simulink model "basicLineFollowing"  (R2016b)
settings: Solver=FixedStepAuto  StartTime=0.0  StopTime=10.0  RelTol=1e-3  EnableMultiTasking=on
undefined symbols (not defined in the file): Comp, Int
libraries: legoev3lib x5
settings Model: ExtModeTrigDuration=2  Creator=Nexel  LastModifiedBy=Nexel
settings SolverCC: PositivePriorityOrder=on
settings OptimizationCC: MaxStackSize=64
settings DebuggingCC: ParameterTunabilityLossMsg=error
settings HardwareCC: ProdBitPerPointer=32  ProdBitPerSizeT=32  ProdBitPerPtrDiffT=32  ProdLargestAtomicInteger=Long  ProdWordSize=32  ProdHWDeviceType=ARM Compatible->ARM 9
settings RTWCC: SystemTargetFile=ert.tlc  HardwareBoard=LEGO MINDSTORMS EV3  TLCOptions="-aInlineSetEventsForThisBaseRateFcn=TLC_FALSE -aSuppressMultiTaskScheduler=TLC_FALSE  -aRateBasedStepFcn=0"  TemplateMakefile=ert_default_tmf  Description=Embedded Coder  GenerateReport=on  Toolchain=Sourcery G++ Lite v2009q3  IncludeHyperlinkInReport=on  LaunchReport=on  GenerateTraceInfo=on  GenerateTraceReport=on  GenerateTraceReportSl=on  GenerateTraceReportSf=on  GenerateTraceReportEml=on
settings CodeAppCC: ForceParamTrailComments=on  IgnoreCustomStorageClasses=off  OperatorAnnotations=on  SimulinkDataObjDesc=on  SFDataObjDesc=on  MATLABFcnDesc=on  InsertBlockDesc=on  MATLABSourceComments=on
settings ERTTargetCC: SupportContinuousTime=on  SupportVariableSizeSignals=on

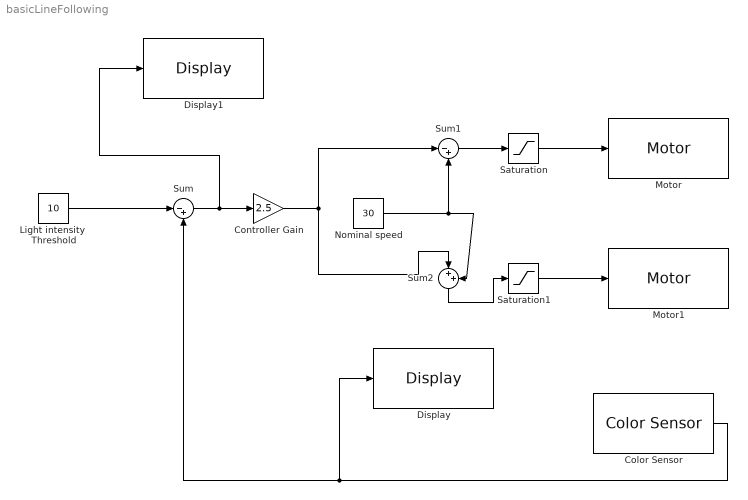
== system basicLineFollowing ==
  Color Sensor : legoev3lib/Color Sensor  portNumber=3  mode=Reflected light intensity  sampleTime=0.1
  "Controller Gain " : Gain  Gain=2.5
  Display : legoev3lib/Display  slcdStr=Int:  slcdLine=2  slcdFormat=Decimal
  Display1 : legoev3lib/Display  slcdStr=Comp:  slcdLine=3  slcdFormat=Decimal
  "Light intensity  Threshold " : Constant  Value=10
  Motor : legoev3lib/Motor  sportNumber=B  sstopAction=Brake
  Motor1 : legoev3lib/Motor  sportNumber=C  sstopAction=Brake
  "Nominal speed " : Constant  Value=30
  Saturation : Saturate  UpperLimit=100  LowerLimit=-100
  Saturation1 : Saturate  UpperLimit=100  LowerLimit=-100
  Sum : Sum  Inputs=|-+
  Sum1 : Sum  Inputs=|-+
  Sum2 : Sum  Inputs=|++
  wires:
  "Light intensity  Threshold "/1 -> Sum/1
  Sum/1 -> Display1/1, "Controller Gain "/1
  Color Sensor/1 -> Display/1, Sum/2
  "Controller Gain "/1 -> Sum2/1, Sum1/1
  "Nominal speed "/1 -> Sum2/2, Sum1/2
  Sum2/1 -> Saturation1/1
  Sum1/1 -> Saturation/1
  Saturation/1 -> Motor/1
  Saturation1/1 -> Motor1/1
